simulink model "smc_simple_rocket"  (R2024a)
settings: Solver=FixedStepAuto  StartTime=0.0  StopTime=20  FixedStep=1e-3  RelTol=1e-3
libraries: aerolibatmos2 x1, aerolibconvert2 x1
settings Model: PacingRate=3  Creator=9310  LastModifiedBy=9310

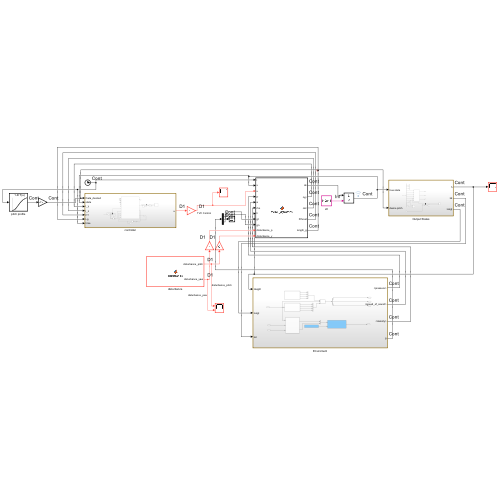
[thumbnail: Simulink's stored preview of the top-level diagram]
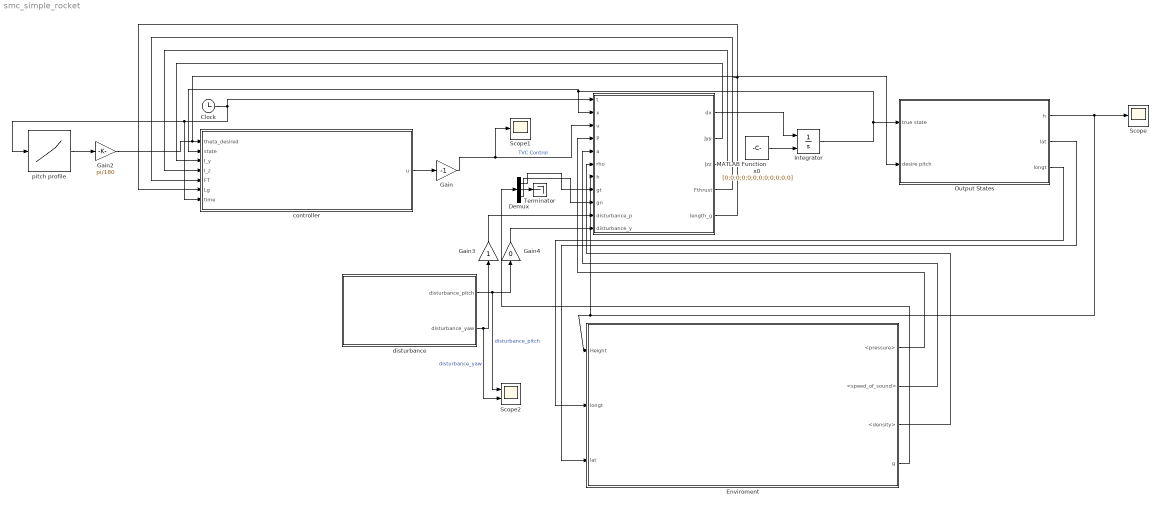
== system smc_simple_rocket ==
  Clock : Clock
  Demux : Demux  Outputs=3
  Enviroment : Subsystem
  Gain : Gain  Gain=-1
  Gain2 : Gain  Gain=pi/180
  Gain3 : Gain
  Gain4 : Gain  Gain=0
  Integrator : Integrator  InitialConditionSource=external
  MATLAB Function : MATLAB Function  TreatAsAtomicUnit=on
  Output States : Subsystem
  Scope : Scope
  Scope1 : Scope
  Scope2 : Scope  NumInputPorts=2
  Terminator : Terminator
  controller : Subsystem
  disturbance : MATLAB Function  TreatAsAtomicUnit=on
  pitch profile : Lookup_n-D  NumberOfTableDimensions=1  BreakpointsForDimension1=[0;1;2;3;4;5;6;7;8;9;10;11;12;13;14;15;16;17;18;19;20;21;22;23;24;25;26;27;28;29;30;31;32;33;34;35;36;37;38;39;40;41;42;43;44;45;46;47;48;49;50;51;52;53;54;55;56;57;58;59;60;61;62;63;64;65;66;67;68;69;70;71;72;73;74;75;76;77;78;79;80;81;82;83;84;85;86;87;88;89;90;91;92;93;94;95;96;97;98;99;100;101;102;103;104;105;106;107;108;109;110;111;112;113;114;115;116;117;118;119;120;121;122;123;124;125;126;127;128;129;130;131;132;133;134;135;136;137;138;139;140]  Table=[0;0;0;0;0;0;0.114095981;0.228191962;0.342287943;0.456383923;0.570479904;0.684575885;0.798671866;0.912767847;1.026863828;1.140959808;1.255055789;1.36915177;1.483247751;1.597343732;1.711439713;2.61563186;2.961557897;3.329942045;3.720405557;4.132495898;4.565700133;5.019449747;5.493122915;5.98605017;6.497520241;7.026785211;7.573065407;8.135553999;8.713424289;9.305841588;9.911959673;10.53092212;11.16186671;11.80392992;12.45624874;13.11797364;13.78826563;14.4662933;15.15123475;15.84228028;16.53864434;17.23960635;17.94455888;18.65292987;19.36418133;20.07781475;20.79335559;21.51035289;22.22846401;22.94749015;23.66726003;24.38762393;25.10833891;25.82914201;26.54970195;27.26959201;27.98841956;28.70595851;29.42174729;30.13511522;30.84522542;31.5515642;32.25368439;32.95113673;33.64351532;34.33041157;35.01143449;35.68625145;36.35450635;37.01591815;37.6701971;38.3170869;38.95637257;39.58782678;40.21129237;40.82658398;41.43358681;42.03216106;42.6222271;43.20368774;43.77649648;44.34059272;44.89596221;45.44251599;45.98013654;46.50883018;47.02865943;47.53966349;48.0419208;48.53549759;49.02047846;49.49695797;49.96502408;50.42478782;50.87635162;51.31982859;51.75533928;52.18301334;52.60303396;53.01553041;53.42062129;53.81843197;54.2090888;54.59271191;54.96942236;55.33934848;55.70261742;56.05935387;56.40968369;56.75373253;57.0916291;57.42349652;57.74945488;58.0696236;58.38412045;58.6930615;58.99656118;59.29473217;59.58768536;59.87553015;60.15837424;60.43632509;60.70949042;60.97797229;61.24187094;61.50128546;61.75631567;62.00705735;62.25360561;62.49605358;62.7344926;62.96901291;63.19970376;63.4266535;63.64994971]  InternalRulePriority=Speed  RndMeth=Simplest
  x0 : Constant  Value=[0;0;0;0;0;0;0;0;0;0;0;0]
  wires:
  MATLAB Function/1(dx) -> Integrator/1
  x0/1 -> Integrator/2
  Clock/1 -> pitch profile/1, controller/7(time), MATLAB Function/1(t)
  disturbance/1(disturbance_pitch) -> Gain4/1, Scope2/1  "disturbance_pitch"
  disturbance/2(disturbance_yaw) -> Gain3/1, Scope2/2  "disturbance_yaw"
  Output States/1(h) -> Scope/1, Enviroment/1(Height), MATLAB Function/7(h)
  Demux/1 -> MATLAB Function/8(gt)
  Demux/3 -> MATLAB Function/9(gn)
  Demux/2 -> Terminator/1
  Enviroment/4(g) -> Demux/1
  Enviroment/1(<pressure>) -> MATLAB Function/4(P)
  Enviroment/2(<speed_of_sound>) -> MATLAB Function/5(a)
  Enviroment/3(<density>) -> MATLAB Function/6(rho)
  Output States/2(lat) -> Enviroment/3(lat)
  Output States/3(longt) -> Enviroment/2(longt)
  Integrator/1 -> MATLAB Function/2(x), controller/2(state), Output States/1(true state)
  Gain3/1 -> MATLAB Function/10(disturbance_p)
  Gain4/1 -> MATLAB Function/11(disturbance_y)
  controller/1(u) -> Gain/1
  MATLAB Function/2(Jyy) -> controller/3(I_y)
  MATLAB Function/3(Jzz) -> controller/4(I_z)
  MATLAB Function/4(Fthrust) -> controller/5(FT)
  MATLAB Function/5(length_g) -> controller/6(Lg)
  Gain/1 -> MATLAB Function/3(u), Scope1/1  "TVC Control"
  pitch profile/1 -> Gain2/1
  Gain2/1 -> Output States/2(desire pitch), controller/1(theta_desired)

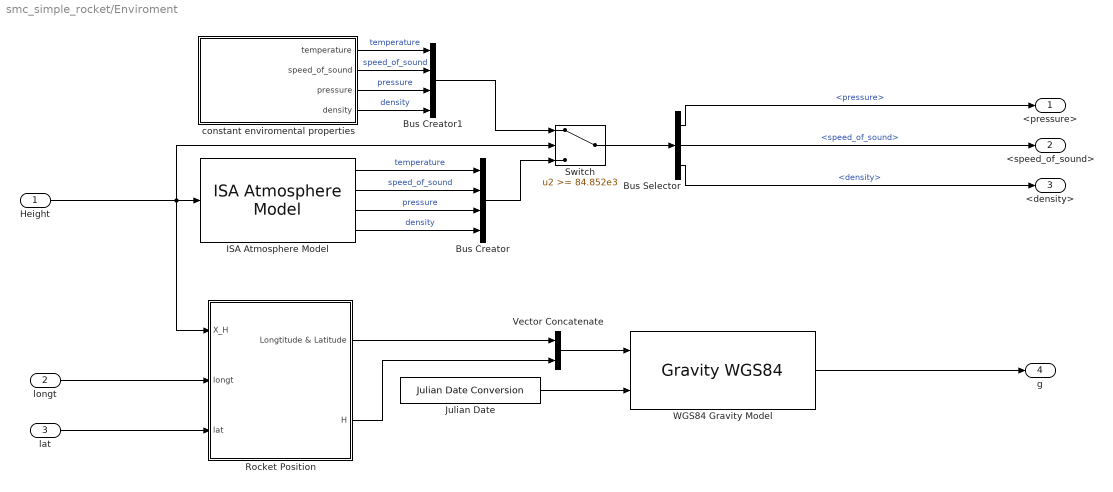
== system smc_simple_rocket/Enviroment ==
  Height : Inport
  longt : Inport  Port=2
  lat : Inport  Port=3
  Bus Creator : BusCreator  Inputs=4
  Bus Creator1 : BusCreator  Inputs=4
  Bus Selector : BusSelector  OutputSignals=pressure,speed_of_sound,density
  ISA Atmosphere Model : aerolibatmos2/ISA Atmosphere Model  useExtended=on  action=None  custom=off  viscosityOut=off  g=9.80665  gamma=1.4  R=287.0531  L=0.0065  h_trop=11000  h_strat=20000  rho0=1.225  P0=101325  T0=288.15  h0=0  S=110.4  Tref=273.15  muref=1.716e-5
  Julian Date : aerolibconvert2/Julian Date Conversion  year=2024  month=July  day=12  hour=11  min=32  sec=3  modflag=off  deltaT=None  errorflag=Error
  Rocket Position : Subsystem
  Switch : Switch  Threshold=84.852e3  SaturateOnIntegerOverflow=off  InputSameDT=off
  Vector Concatenate : Concatenate
  "WGS84 Gravity Model  " : GravityWGS84  model=WGS84 Exact  jd_loc=on  no_centrifugal=off  action=None
  "constant enviromental properties " : Subsystem
  <pressure> : Outport
  <speed_of_sound> : Outport  Port=2
  <density> : Outport  Port=3
  g : Outport  Port=4
  wires:
  "constant enviromental properties "/4(density) -> Bus Creator1/4  "density"
  Bus Creator1/1 -> Switch/1
  Bus Creator/1 -> Switch/3
  ISA Atmosphere Model/4 -> Bus Creator/4  "density"
  "constant enviromental properties "/2(speed_of_sound) -> Bus Creator1/2  "speed_of_sound"
  ISA Atmosphere Model/3 -> Bus Creator/3  "pressure"
  ISA Atmosphere Model/1 -> Bus Creator/1  "temperature"
  ISA Atmosphere Model/2 -> Bus Creator/2  "speed_of_sound"
  "constant enviromental properties "/1(temperature) -> Bus Creator1/1  "temperature"
  "constant enviromental properties "/3(pressure) -> Bus Creator1/3  "pressure"
  Height/1 -> Switch/2, ISA Atmosphere Model/1, Rocket Position/1(X_H)
  Switch/1 -> Bus Selector/1
  Bus Selector/1 -> <pressure>/1  "<pressure>"
  Julian Date/1 -> "WGS84 Gravity Model  "/2
  Rocket Position/1(Longtitude & Latitude) -> Vector Concatenate/1
  Rocket Position/2(H) -> Vector Concatenate/2
  Vector Concatenate/1 -> "WGS84 Gravity Model  "/1
  "WGS84 Gravity Model  "/1 -> g/1
  Bus Selector/2 -> <speed_of_sound>/1  "<speed_of_sound>"
  Bus Selector/3 -> <density>/1  "<density>"
  longt/1 -> Rocket Position/2(longt)
  lat/1 -> Rocket Position/3(lat)

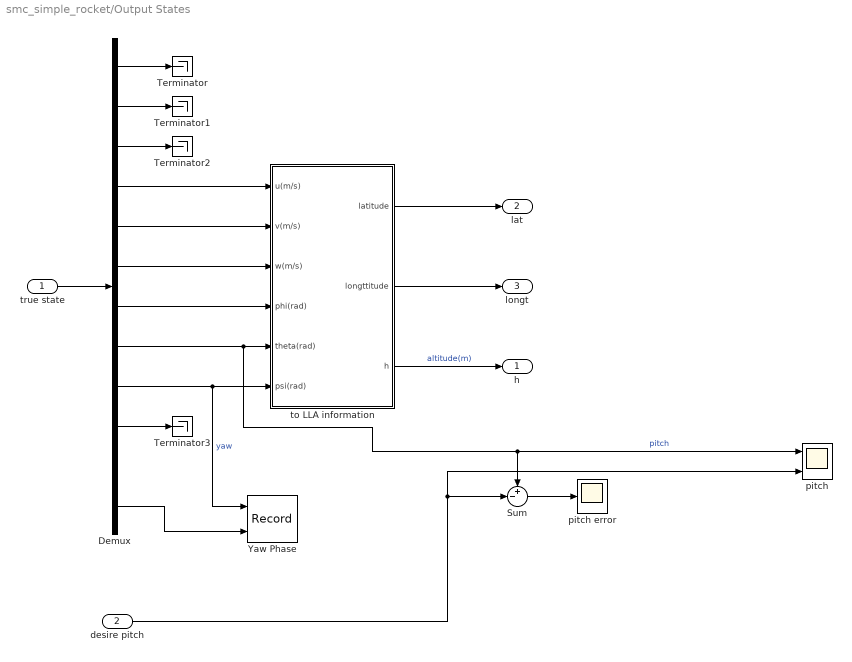
== system smc_simple_rocket/Output States ==
  true state : Inport
  desire pitch : Inport  Port=2
  Demux : Demux  Outputs=12
  Sum : Sum  Inputs=+-|
  Terminator{,1..3} (4 alike) : Terminator
  Yaw Phase : Record  FileSettingsInternal="{\"entries\":[{\"content\":{\"excelSettings\":{\"content\":{},\"type\":\"Streamout.ExcelSettings\"}},\"type\":\"Streamout.FileSettingStorage\",\"uuid\":\"\"}],\"packageUris\":[\"http:\\/\\/schema.mathworks.com\\/mf0\\/streamout_blocks\\/R2020a\"],\"version\":\"1.0\"}"  Layout=[1 1]  SignalsInternal="{\"entries\":[{\"content\":{\"signals\":[{\"content\":{\"blockPath\":[],\"dimensions\":[1],\"domain\":\"\",\"lineColor\":\"#64d413\",\"lineWidth\":2,\"port\":1,\"sid\":[\"\"],\"signalID\":1,\"signalName\":\"yaw\"},\"type\":\"RecordBlkView.Signal\",\"uuid\":\"\"},{\"content\":{\"blockPath\":[],\"dimensions\":[1],\"domain\":\"\",\"lineColor\":\"#ff13a6\",\"lineWidth\":2,\"port\":2,\"sid\":[\"\"],\"signalID\":2,\"signalName\":\"Demux:12\"},\"type\":\"RecordBlkView.Signal\",\"uuid\":\"\"}]},\"type\":\"RecordBlkView.InputSignals\",\"uuid\":\"\"}],\"packageUris\":[\"http:\\/\\/schema.mathworks.com\\/mf0\\/streamout_blocks\\/R2020a\"],\"version\":\"1.0\"}"  VisualizationBindings="{\"xyplotplugin\":{\"info\":[{\"series\":[],\"subplotID\":1}]}}"  CompatibilityTag=XY
  pitch : Scope  NumInputPorts=2
  pitch error : Scope
  to LLA information : Subsystem
  h : Outport
  lat : Outport  Port=2
  longt : Outport  Port=3
  wires:
  true state/1 -> Demux/1
  Demux/1 -> Terminator/1
  Demux/2 -> Terminator1/1
  Demux/3 -> Terminator2/1
  Demux/4 -> to LLA information/1(u(m/s))
  Demux/5 -> to LLA information/2(v(m/s))
  Demux/6 -> to LLA information/3(w(m/s))
  Demux/7 -> to LLA information/4(phi(rad))
  Demux/8 -> Sum/1, pitch/1, to LLA information/5(theta(rad))  "pitch"
  Demux/9 -> to LLA information/6(psi(rad)), Yaw Phase/1  "yaw"
  to LLA information/3(h) -> h/1  "altitude(m)"
  to LLA information/2(longttitude) -> longt/1
  to LLA information/1(latitude) -> lat/1
  Demux/10 -> Terminator3/1
  Demux/12 -> Yaw Phase/2
  desire pitch/1 -> pitch/2, Sum/2
  Sum/1 -> pitch error/1

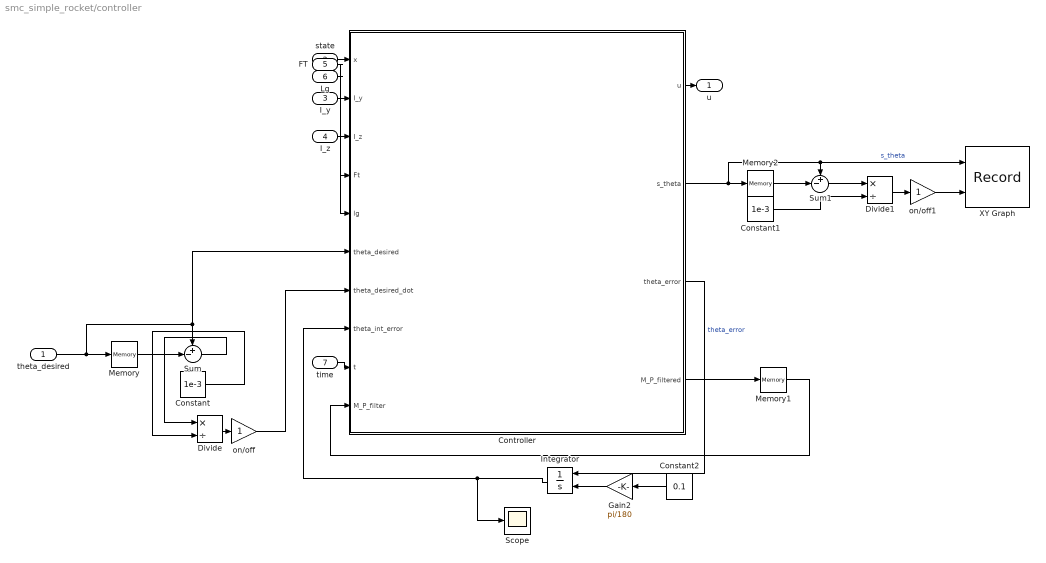
== system smc_simple_rocket/controller ==
  theta_desired : Inport
  state : Inport  Port=2
  I_y : Inport  Port=3
  I_z : Inport  Port=4
  FT : Inport  Port=5
  Lg : Inport  Port=6
  time : Inport  Port=7
  Constant : Constant  Value=1e-3
  Constant1 : Constant  Value=1e-3
  Constant2 : Constant  Value=0.1
  Controller : MATLAB Function  TreatAsAtomicUnit=on
  Divide : Product  Inputs=*/
  Divide1 : Product  Inputs=*/
  Gain2 : Gain  Gain=pi/180
  Integrator : Integrator  InitialConditionSource=external
  Memory : Memory  InheritSampleTime=on
  Memory1 : Memory
  Memory2 : Memory
  Scope : Scope
  Sum : Sum  Inputs=+-|
  Sum1 : Sum  Inputs=+-|
  XY Graph : Record  FileSettingsInternal="{\"entries\":[{\"content\":{\"excelSettings\":{\"content\":{},\"type\":\"Streamout.ExcelSettings\"}},\"type\":\"Streamout.FileSettingStorage\",\"uuid\":\"\"}],\"packageUris\":[\"http:\\/\\/schema.mathworks.com\\/mf0\\/streamout_blocks\\/R2020a\"],\"version\":\"1.0\"}"  Layout=[1 1]  SignalsInternal="{\"entries\":[{\"content\":{\"signals\":[{\"content\":{\"blockPath\":[],\"dimensions\":[1],\"domain\":\"\",\"lineColor\":\"#a2142f\",\"plots\":[ 1 ],\"port\":1,\"sid\":[\"\"],\"signalID\":1,\"signalName\":\"s_theta\"},\"type\":\"RecordBlkView.Signal\",\"uuid\":\"\"},{\"content\":{\"blockPath\":[],\"dimensions\":[1],\"domain\":\"\",\"lineColor\":\"#139fff\",\"plots\":[ 1 ],\"port\":2,\"sid\":[\"\"],\"signalID\":2,\"signalName\":\"on\\/off1\"},\"type\":\"RecordBlkView.Signal\",\"uuid\":\"\"}]},\"type\":\"RecordBlkView.InputSignals\",\"uuid\":\"\"}],\"packageUris\":[\"http:\\/\\/schema.mathworks.com\\/mf0\\/streamout_blocks\\/R2020a\"],\"version\":\"1.0\"}"  VisualizationBindings="{\"xyplotplugin\":{\"info\":[{\"series\":[{\"bindingParametersList\":[{\"parameter\":\"X-Axis\",\"signalID\":1,\"signalName\":\"s_theta\"},{\"parameter\":\"Y-Axis\",\"signalID\":2,\"signalName\":\"on\\/off1\"}],\"seriesID\":0}],\"subplotID\":1}]}}"  CompatibilityTag=XY
  on/off : Gain
  on/off1 : Gain
  u : Outport
  wires:
  Memory/1 -> Sum/2
  Divide/1 -> on/off/1
  Constant/1 -> Divide/2
  Sum/1 -> Divide/1
  theta_desired/1 -> Sum/1, Controller/6(theta_desired), Memory/1
  state/1 -> Controller/1(x)
  FT/1 -> Controller/4(Ft)
  I_y/1 -> Controller/2(I_y)
  I_z/1 -> Controller/3(I_z)
  Lg/1 -> Controller/5(lg)
  Controller/1(u) -> u/1
  on/off/1 -> Controller/7(theta_desired_dot)
  Controller/3(theta_error) -> Integrator/1  "theta_error"
  Integrator/1 -> Scope/1, Controller/8(theta_int_error)
  time/1 -> Controller/9(t)
  Controller/4(M_P_filtered) -> Memory1/1
  Memory1/1 -> Controller/10(M_P_filter)
  Controller/2(s_theta) -> XY Graph/1, Sum1/1, Memory2/1  "s_theta"
  Memory2/1 -> Sum1/2
  Sum1/1 -> Divide1/1
  Constant1/1 -> Divide1/2
  Divide1/1 -> on/off1/1
  on/off1/1 -> XY Graph/2
  Gain2/1 -> Integrator/2
  Constant2/1 -> Gain2/1

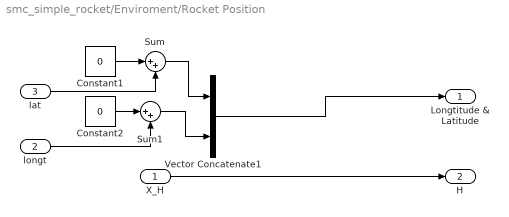
== system smc_simple_rocket/Enviroment/Rocket Position ==
  X_H : Inport
  longt : Inport  Port=2
  lat : Inport  Port=3
  Constant1 : Constant  Value=0
  Constant2 : Constant  Value=0
  Sum : Sum  Inputs=|++
  Sum1 : Sum  Inputs=|++
  Vector Concatenate1 : Concatenate
  Longtitude & Latitude : Outport
  H : Outport  Port=2
  wires:
  Vector Concatenate1/1 -> Longtitude & Latitude/1
  X_H/1 -> H/1
  Constant1/1 -> Sum/1
  Constant2/1 -> Sum1/1
  Sum/1 -> Vector Concatenate1/1
  Sum1/1 -> Vector Concatenate1/2
  lat/1 -> Sum/2
  longt/1 -> Sum1/2

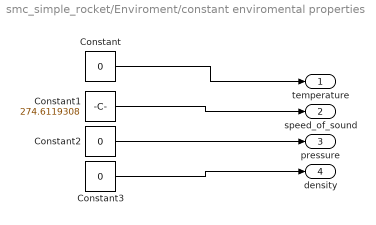
== system smc_simple_rocket/Enviroment/constant enviromental properties  ==
  Constant : Constant  Value=0
  Constant1 : Constant  Value=274.6119308
  Constant2 : Constant  Value=0
  Constant3 : Constant  Value=0
  temperature : Outport
  speed_of_sound : Outport  Port=2
  pressure : Outport  Port=3
  density : Outport  Port=4
  wires:
  Constant/1 -> temperature/1
  Constant1/1 -> speed_of_sound/1
  Constant2/1 -> pressure/1
  Constant3/1 -> density/1

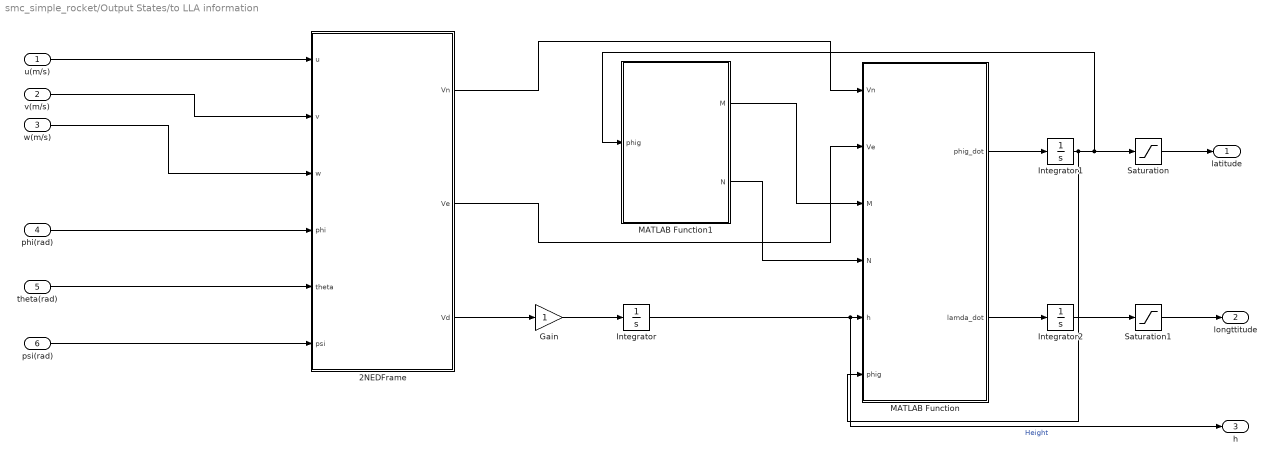
== system smc_simple_rocket/Output States/to LLA information ==
  u(m/s) : Inport
  v(m/s) : Inport  Port=2
  w(m/s) : Inport  Port=3
  phi(rad) : Inport  Port=4
  theta(rad) : Inport  Port=5
  psi(rad) : Inport  Port=6
  2NEDFrame : MATLAB Function  TreatAsAtomicUnit=on
  Gain : Gain
  Integrator : Integrator
  Integrator1 : Integrator
  Integrator2 : Integrator
  MATLAB Function : MATLAB Function  TreatAsAtomicUnit=on
  MATLAB Function1 : MATLAB Function  TreatAsAtomicUnit=on
  Saturation : Saturate  UpperLimit=pi/2  LowerLimit=-pi/2
  Saturation1 : Saturate  UpperLimit=pi  LowerLimit=-pi
  latitude : Outport
  longttitude : Outport  Port=2
  h : Outport  Port=3
  wires:
  u(m/s)/1 -> 2NEDFrame/1(u)
  v(m/s)/1 -> 2NEDFrame/2(v)
  w(m/s)/1 -> 2NEDFrame/3(w)
  phi(rad)/1 -> 2NEDFrame/4(phi)
  psi(rad)/1 -> 2NEDFrame/6(psi)
  theta(rad)/1 -> 2NEDFrame/5(theta)
  2NEDFrame/3(Vd) -> Gain/1
  Gain/1 -> Integrator/1
  Integrator/1 -> h/1, MATLAB Function/5(h)  "Height"
  MATLAB Function1/1(M) -> MATLAB Function/3(M)
  MATLAB Function1/2(N) -> MATLAB Function/4(N)
  2NEDFrame/1(Vn) -> MATLAB Function/1(Vn)
  2NEDFrame/2(Ve) -> MATLAB Function/2(Ve)
  MATLAB Function/1(phig_dot) -> Integrator1/1
  MATLAB Function/2(lamda_dot) -> Integrator2/1
  Integrator1/1 -> MATLAB Function/6(phig), Saturation/1, MATLAB Function1/1(phig)
  Integrator2/1 -> Saturation1/1
  Saturation/1 -> latitude/1
  Saturation1/1 -> longttitude/1

== matlab function smc_simple_rocket/Output States/to LLA information/2NEDFrame ==
  data: u input; Vn output; v input; w input; phi input; theta input; psi input; Ve output; Vd output
function [Vn, Ve, Vd] = navigation_equations(u, v, w, phi, theta, psi)
    % Calculate transformation matrix components
    R11 = cos(theta) * cos(psi);
    R12 = cos(theta) * sin(psi);
    R13 = -sin(theta);
    R21 = sin(phi) * sin(theta) * cos(psi) - cos(phi) * sin(psi);
    R22 = sin(phi) * sin(theta) * sin(psi) + cos(phi) * cos(psi);
    R23 = sin(phi) * cos(theta);
    R31 = cos(phi) * sin(theta) * cos(psi) + sin(phi) * sin(psi);
    R32 = cos(phi) * sin(theta) * sin(psi) - sin(phi) * cos(psi);
    R33 = cos(phi) * cos(theta);
    
    % Transform body velocities to navigation frame
    Vn = R31 * u + R32 * v + R33 * w;
    Ve = R21 * u + R22 * v + R23 * w;
    Vd = R11 * u + R12 * v + R13 * w;
end

== matlab function smc_simple_rocket/Output States/to LLA information/MATLAB Function ==
  data: Vn input; phig_dot output; Ve input; M input; N input; h input; phig input; lamda_dot output
function [phig_dot,lamda_dot] = fcn(Vn,Ve,M,N,h,phig)

phig_dot = Vn / (M+h);
lamda_dot = Ve / ((N+h)*cos(phig));

== matlab function smc_simple_rocket/Output States/to LLA information/MATLAB Function1 ==
  data: phig input; M output; N output
function [M,N] = WGS84(phig)

a = 6378137; % Equitorial Radius
ec = 0.081819190842622; % First Eccentricity
M = (a*(1-ec^2))/((1-(ec^2)*(sin(phig)^2))^(3/2)); % Meridian Radius
N = (a)/(sqrt(1-((ec^2)*(sin(phig)^2))));

== matlab function smc_simple_rocket/controller/Controller ==
  settings: updateMethod=DISCRETE
  data: x input; I_y input; I_z input; Ft input; lg input; u output; s_theta output; theta_desired input; theta_desired_dot input; theta_error output; theta_int_error input; t input; M_P_filter input; M_P_filtered output
function [u,s_theta,theta_error,M_P_filtered]= Improved_SMC_control(x, I_y, I_z, Ft, lg, theta_desired, theta_desired_dot, theta_int_error,t,M_P_filter)
    % State variables
    phi = x(7);
    theta = x(8);
    psi = x(9);
    omega = x(10:12);
    theta_dot = cos(phi)*omega(2)-sin(phi)*omega(3);
    psi_dot = omega(3);

    % SMC parameters
    lambda_theta = 5;  % P
    lambda_psi = 5;
    lambda_theta_int = 4; % I
    lambda_psi_int = 4;
    lambda_theta_dot = 1.2; % D
    lambda_psi_dot = 0.8;
    K_theta = 1.5 * I_y; 
    K_psi = I_z;
    c_theta = 4 * K_theta;  % Increased Ftom 3*K_theta
    c_psi = 3 * K_psi;
    K_nl = 10 * K_theta;

    % Calculate pitch error and its derivative
    theta_error = theta - theta_desired;
    theta_dot_error = theta_dot - theta_desired_dot;

    % Sliding surfaces
    % Time-varying sliding surface
    alpha = 0.35*t;
    s_theta = lambda_theta_dot*theta_dot_error + lambda_theta * theta_error + alpha* lambda_theta_int * theta_int_error;
    s_psi = lambda_psi_dot*psi_dot + lambda_psi * psi;

    % Replace the sat function with a continuous approximation
    s_theta_normalized = (s_theta/0.001);
    sat_approx = s_theta_normalized / (1 + abs(s_theta_normalized));
    
    % Nonlinear damping term
    nonlinear_damping = K_nl * sqrt(abs(s_theta)) * sat_approx; 

    % Control law with feedforward term
    M_P = -K_theta * sat_approx - c_theta * s_theta - nonlinear_damping;
    M_Y = -K_psi * sat_approx - c_psi * s_psi;
    
    %Super-Twisting parameters
    % alpha = 0.1* sqrt(2 * K_theta);
    % beta = 0.1 * K_theta;
    % dz = beta * sat_approx;
    % z = z_p + dz * 0.001;
    % M_P = -alpha * sqrt(abs(s_theta)) * sat_approx - z;

    if isempty(M_P_filter)
        M_P_filter = M_P;
    end
    alpha_filter = 0.4;  % Assuming 0.01s sample time
    M_P_filtered = alpha_filter * M_P_filter + (1 - alpha_filter) * M_P;

    % TVC angle command
    % Calculate deltaY
    sin_deltaY = M_Y / (Ft * lg);
    sin_deltaY = min(max(sin_deltaY, -1), 1);
    deltaY = asin(sin_deltaY);
    
    % Calculate deltaP
    cos_deltaY = sqrt(1 - sin_deltaY^2);
    sin_deltaP = M_P_filtered / (-Ft * lg * cos_deltaY);
    sin_deltaP = min(max(sin_deltaP, -1), 1);
    deltaP = asin(sin_deltaP);
    

    % Return control inputs
    u = [deltaY; deltaP];
end

== matlab function smc_simple_rocket/MATLAB Function ==
  data: dx output size=12; Jyy output size=1; Jzz output size=1; Fthrust output size=1; t input; x input; u input; P input; a input; rho input; h input; gt input; gn input; disturbance_p input; length_g output size=1; disturbance_y input
% Function definition for Simulink MATLAB Function Block
function [dx, Jyy, Jzz, Fthrust, length_g] = rocket_dynamics(t, x, u, P, a, rho, h, gt, gn, disturbance_p, disturbance_y)
% Define output dimensions for Simulink
%#codegen

% Preallocate outputs with known dimensions
dx = zeros(12, 1);
Jyy = 0;
Jzz = 0;
Fthrust = 0;
length_g = 0;


% Call the original function
[dx, Jyy, Jzz, Fthrust, length_g] = six_dof_rocket_sim(t, x, u, P, a, rho, h, gt, gn, disturbance_p, disturbance_y);

% Ensure all outputs are at least scalar (1x1)
Jyy = double(Jyy);
Jzz = double(Jzz);
Fthrust = double(Fthrust);
length_g = double(length_g);
end

== matlab function smc_simple_rocket/disturbance ==
  settings: updateMethod=DISCRETE
  data: disturbance_pitch output; disturbance_yaw output
function [disturbance_pitch, disturbance_yaw] = disturbance()
        disturbance_pitch =  12 * randn; % Constant with noise
        disturbance_yaw = 5 * randn; % Constant with noise
end
